simulink model "Vertikaler_Wurf"  (R2025b)
settings: Solver=VariableStepAuto  StartTime=0.0  StopTime=10.0  RelTol=1e-3
settings Model: Creator=georg  LastModifiedBy=georg

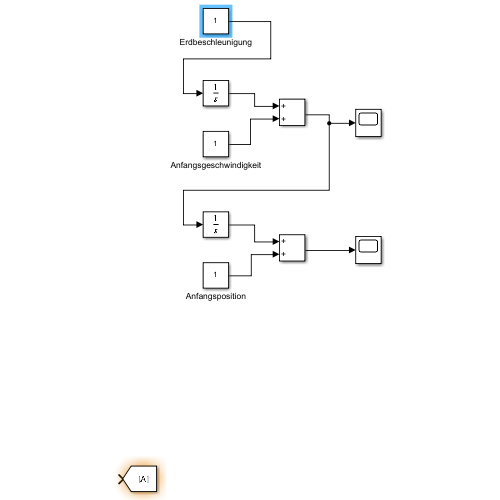
[thumbnail: Simulink's stored preview of the top-level diagram]
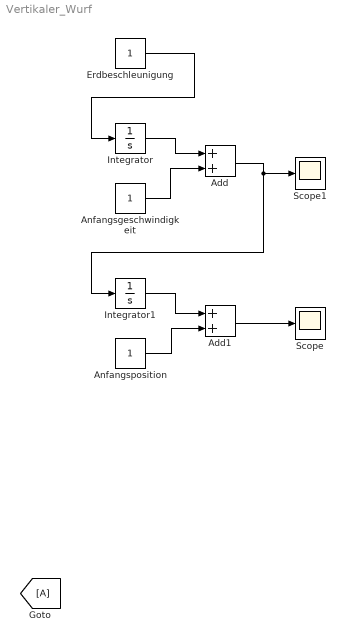
== system Vertikaler_Wurf ==
  Add : Sum
  Add1 : Sum
  Anfangsgeschwindigkeit : Constant
  Anfangsposition : Constant
  Erdbeschleunigung : Constant
  Goto : Goto
  Integrator : Integrator
  Integrator1 : Integrator
  Scope : Scope
  Scope1 : Scope
  wires:
  Erdbeschleunigung/1 -> Integrator/1
  Integrator/1 -> Add/1
  Anfangsgeschwindigkeit/1 -> Add/2
  Add/1 -> Integrator1/1, Scope1/1
  Integrator1/1 -> Add1/1
  Anfangsposition/1 -> Add1/2
  Add1/1 -> Scope/1
